simulink model "mrefrobotarm_modified_previous_y_previous_u_previous_ref_prepro"  (R2018b)
settings: Solver=FixedStepAuto  StartTime=0.0  StopTime=10  RelTol=1e-3  AbsTol=1e-6
undefined symbols (not defined in the file or in its folder): cc, options
libraries: neural x594, simulink x1
(part 16 of 22)

== system mrefrobotarm_modified_previous_y_previous_u_previous_ref_prepro/pre_0.00004/Layer 3/Delays 1 ==
  "p{3}" : Inport  PortDimensions=30
      mask Display: e = 0.06;c1 = [120 230 180]/255;c2 = ([120 230 180]+0)/(256+128);c3 = ([120 230 180]+128)/(256+128);patch([0 1 1 0],[0 0 1 1],c1);patch([0 1 1 1-e 1-e 0+e],[0 0 1 1-e 0+e 0+e],c2);patch([0 0 1 1-e 0+e 0+e],[0 1 1 1-e 1-e 0+e],c3);plot([0 1 1 0 0],[0 0 1 1 0]);
  mux : Mux  Inputs=1
      mask Display: e = 0.06;c1 = [120 150 230]/255;c2 = ([120 150 230]+0)/383;c3 = ([120 150 230]+128)/383;patch([0 1 1 0],[0 0 1 1],c1);patch([0 1 1 1-e 1-e 0+e],[0 0 1 1-e 0+e 0+e],c2);patch([0 0 1 1-e 0+e 0+e],[0 1 1 1-e 1-e 0+e],c3);plot([0 1 1 0 0],[0 0 1 1 0]);disp('Mux')
  "pd{3,2}" : Outport
      mask Display: e = 0.06;c1 = [120 230 180]/255;c2 = ([120 230 180]+0)/(256+128);c3 = ([120 230 180]+128)/(256+128);patch([0 1 1 0],[0 0 1 1],c1);patch([0 1 1 1-e 1-e 0+e],[0 0 1 1-e 0+e 0+e],c2);patch([0 0 1 1-e 0+e 0+e],[0 1 1 1-e 1-e 0+e],c3);plot([0 1 1 0 0],[0 0 1 1 0]);
  wires:
  "p{3}"/1 -> mux/1
  mux/1 -> "pd{3,2}"/1

== system mrefrobotarm_modified_previous_y_previous_u_previous_ref_prepro/pre_0.00004/Layer 3/LW{3,2} ==
  "ad{3,2}" : Inport  PortDimensions=30
      mask Display: e = 0.06;c1 = [120 230 180]/255;c2 = ([120 230 180]+0)/(256+128);c3 = ([120 230 180]+128)/(256+128);patch([0 1 1 0],[0 0 1 1],c1);patch([0 1 1 1-e 1-e 0+e],[0 0 1 1-e 0+e 0+e],c2);patch([0 0 1 1-e 0+e 0+e],[0 1 1 1-e 1-e 0+e],c3);plot([0 1 1 0 0],[0 0 1 1 0]);
  "IW{3,2}(1,:)'" : Constant  Value=[-0.12115323977208213024336913576917140744626522064208984375;0.1421645828481130913178986929779057390987873077392578125;0.2104360456092702891250922903054743073880672454833984375;-0.209627821379691436920467140225809998810291290283203125;0.399324974589913506139993160104495473206043243408203125;0.5108287033332643556349239588598720729351043701171875;-0.01755690203553068873265630145397153683006763458251953125;-0.398676925843608864763467636294080875813961029052734375;0.00184641474824170752355723124082942376844584941864013671875;0.267730388383461248569261670127161778509616851806640625;-0.2285341543329846292209595048916526138782501220703125;-0.14635003276886104917053899043821729719638824462890625;-0.290530902647844369024454636019072495400905609130859375;-0.18623054223144297480985187576152384281158447265625;-0.3816641765859636326041481879656203091144561767578125;0.422608587689044135071725349916960112750530242919921875;-0.50402602801203333360291480857995338737964630126953125;0.04787057638839231632488235845812596380710601806640625;0.26072024791618420014316370725282467901706695556640625;0.03130735790264956019957054422775399871170520782470703125;-0.184803625769296819836284839766449294984340667724609375;-0.07897098331966272144466501003989833407104015350341796875;0.318614464740402614228997890677419491112232208251953125;-0.32476411310026553902474688584334217011928558349609375;0.31226160654872237021351111252442933619022369384765625;0.08174671514652807891021524255847907625138759613037109375;-0.289500256123392085694234765469445846974849700927734375;-0.2644913786315357118184010687400586903095245361328125;0.06532576379320138848516563712109928019344806671142578125;0.088750906118596761817940432592877186834812164306640625]
      mask Display: e = 0.06;c1 = [120 150 230]/255;c2 = ([120 150 230]+0)/383;c3 = ([120 150 230]+128)/383;patch([0 1 1 0],[0 0 1 1],c1);patch([0 1 1 1-e 1-e 0+e],[0 0 1 1-e 0+e 0+e],c2);patch([0 0 1 1-e 0+e 0+e],[0 1 1 1-e 1-e 0+e],c3);plot([0 1 1 0 0],[0 0 1 1 0]);disp('weights');
  Mux : Mux  Inputs=1
      mask Display: e = 0.06;c1 = [120 150 230]/255;c2 = ([120 150 230]+0)/383;c3 = ([120 150 230]+128)/383;patch([0 1 1 0],[0 0 1 1],c1);patch([0 1 1 1-e 1-e 0+e],[0 0 1 1-e 0+e 0+e],c2);patch([0 0 1 1-e 0+e 0+e],[0 1 1 1-e 1-e 0+e],c3);plot([0 1 1 0 0],[0 0 1 1 0]);disp('Mux');
  dotprod1 : neural/Weight Functions/dotprod
  "lz{3,2}" : Outport
      mask Display: e = 0.06;c1 = [120 230 180]/255;c2 = ([120 230 180]+0)/(256+128);c3 = ([120 230 180]+128)/(256+128);patch([0 1 1 0],[0 0 1 1],c1);patch([0 1 1 1-e 1-e 0+e],[0 0 1 1-e 0+e 0+e],c2);patch([0 0 1 1-e 0+e 0+e],[0 1 1 1-e 1-e 0+e],c3);plot([0 1 1 0 0],[0 0 1 1 0]);
  wires:
  "IW{3,2}(1,:)'"/1 -> dotprod1/1
  "ad{3,2}"/1 -> dotprod1/2
  dotprod1/1 -> Mux/1
  Mux/1 -> "lz{3,2}"/1

== system mrefrobotarm_modified_previous_y_previous_u_previous_ref_prepro/pre_0.0001/Layer 1/Delays 1 ==
  "p{1}" : Inport  PortDimensions=10
      mask Display: e = 0.06;c1 = [120 230 180]/255;c2 = ([120 230 180]+0)/(256+128);c3 = ([120 230 180]+128)/(256+128);patch([0 1 1 0],[0 0 1 1],c1);patch([0 1 1 1-e 1-e 0+e],[0 0 1 1-e 0+e 0+e],c2);patch([0 0 1 1-e 0+e 0+e],[0 1 1 1-e 1-e 0+e],c3);plot([0 1 1 0 0],[0 0 1 1 0]);
  mux : Mux  Inputs=1
      mask Display: e = 0.06;c1 = [120 150 230]/255;c2 = ([120 150 230]+0)/383;c3 = ([120 150 230]+128)/383;patch([0 1 1 0],[0 0 1 1],c1);patch([0 1 1 1-e 1-e 0+e],[0 0 1 1-e 0+e 0+e],c2);patch([0 0 1 1-e 0+e 0+e],[0 1 1 1-e 1-e 0+e],c3);plot([0 1 1 0 0],[0 0 1 1 0]);disp('Mux')
  "pd{1,1}" : Outport
      mask Display: e = 0.06;c1 = [120 230 180]/255;c2 = ([120 230 180]+0)/(256+128);c3 = ([120 230 180]+128)/(256+128);patch([0 1 1 0],[0 0 1 1],c1);patch([0 1 1 1-e 1-e 0+e],[0 0 1 1-e 0+e 0+e],c2);patch([0 0 1 1-e 0+e 0+e],[0 1 1 1-e 1-e 0+e],c3);plot([0 1 1 0 0],[0 0 1 1 0]);
  wires:
  "p{1}"/1 -> mux/1
  mux/1 -> "pd{1,1}"/1

== system mrefrobotarm_modified_previous_y_previous_u_previous_ref_prepro/pre_0.0001/Layer 1/IW{1,1} ==
  "pd{1,1}" : Inport  PortDimensions=10
      mask Display: e = 0.06;c1 = [120 230 180]/255;c2 = ([120 230 180]+0)/(256+128);c3 = ([120 230 180]+128)/(256+128);patch([0 1 1 0],[0 0 1 1],c1);patch([0 1 1 1-e 1-e 0+e],[0 0 1 1-e 0+e 0+e],c2);patch([0 0 1 1-e 0+e 0+e],[0 1 1 1-e 1-e 0+e],c3);plot([0 1 1 0 0],[0 0 1 1 0]);
  "IW{1,1}(1,:)'" : Constant  Value=[0.48848188030832784267687429746729321777820587158203125;-0.50670985753113895189159165965975262224674224853515625;0.10409356491148090417819815911570913158357143402099609375;0.225809349826792404858366580810979939997196197509765625;0.4009865161841350555960161727853119373321533203125;0.169825092265467658680933027426362968981266021728515625;0.78830762047560887229025183842168189585208892822265625;0.8853776813051636995766102700144983828067779541015625;-1.267910607500292829996624277555383741855621337890625;-0.31884147881028657156576855413732118904590606689453125]
      mask Display: e = 0.06;c1 = [120 150 230]/255;c2 = ([120 150 230]+0)/383;c3 = ([120 150 230]+128)/383;patch([0 1 1 0],[0 0 1 1],c1);patch([0 1 1 1-e 1-e 0+e],[0 0 1 1-e 0+e 0+e],c2);patch([0 0 1 1-e 0+e 0+e],[0 1 1 1-e 1-e 0+e],c3);plot([0 1 1 0 0],[0 0 1 1 0]);disp('Weights');
  "IW{1,1}(10,:)'" : Constant  Value=[0.60982224497398618279220272597740404307842254638671875;-0.93656291188809603909248835407197475433349609375;0.0979830538632104619534146650039474479854106903076171875;-0.87957865814192859321707373965182341635227203369140625;-0.30231253806006563866759506709058769047260284423828125;0.199503786892032464184154605391086079180240631103515625;-1.1899431974826459867955463778343982994556427001953125;-0.03266430327928458721142845888607553206384181976318359375;0.3019162611871599732893400869215838611125946044921875;0.1610107886790740627791507222354994155466556549072265625]
      mask Display: e = 0.06;c1 = [120 150 230]/255;c2 = ([120 150 230]+0)/383;c3 = ([120 150 230]+128)/383;patch([0 1 1 0],[0 0 1 1],c1);patch([0 1 1 1-e 1-e 0+e],[0 0 1 1-e 0+e 0+e],c2);patch([0 0 1 1-e 0+e 0+e],[0 1 1 1-e 1-e 0+e],c3);plot([0 1 1 0 0],[0 0 1 1 0]);disp('Weights');
  "IW{1,1}(11,:)'" : Constant  Value=[0.43117720603294940051597450292319990694522857666015625;-1.1157191661762866363716284467955119907855987548828125;0.3922109909243991499039339032606221735477447509765625;-0.496959837462516540451673563438816927373409271240234375;0.01695143984838747008847548158883000724017620086669921875;1.3205255898856946839003967397729866206645965576171875;0.02046825294557734487010947077578748576343059539794921875;-0.346542077133276948952556040239869616925716400146484375;-0.87405349501553997182412558686337433755397796630859375;0.49868545376052519912946081603877246379852294921875]
      mask Display: e = 0.06;c1 = [120 150 230]/255;c2 = ([120 150 230]+0)/383;c3 = ([120 150 230]+128)/383;patch([0 1 1 0],[0 0 1 1],c1);patch([0 1 1 1-e 1-e 0+e],[0 0 1 1-e 0+e 0+e],c2);patch([0 0 1 1-e 0+e 0+e],[0 1 1 1-e 1-e 0+e],c3);plot([0 1 1 0 0],[0 0 1 1 0]);disp('Weights');
  "IW{1,1}(12,:)'" : Constant  Value=[-0.545805604712654268695359860430471599102020263671875;-0.65828716083673766146233674589893780648708343505859375;-0.04018956631550653357809466115213581360876560211181640625;0.06817452770580727239302376574414665810763835906982421875;-0.812439650403700586167587971431203186511993408203125;-0.15845568778963892153655024230829440057277679443359375;-0.345942575000688201658505249724839814007282257080078125;-0.1536078830084397217614622377368505112826824188232421875;-0.9507981209733535887806965547497384250164031982421875;-0.93008098611112532960731869025039486587047576904296875]
      mask Display: e = 0.06;c1 = [120 150 230]/255;c2 = ([120 150 230]+0)/383;c3 = ([120 150 230]+128)/383;patch([0 1 1 0],[0 0 1 1],c1);patch([0 1 1 1-e 1-e 0+e],[0 0 1 1-e 0+e 0+e],c2);patch([0 0 1 1-e 0+e 0+e],[0 1 1 1-e 1-e 0+e],c3);plot([0 1 1 0 0],[0 0 1 1 0]);disp('Weights');
  "IW{1,1}(13,:)'" : Constant  Value=[0.66295360405807157722080091843963600695133209228515625;-0.8938461691272043818656811708933673799037933349609375;-0.307383457603058740659207614953629672527313232421875;0.7696942151114913865939115567016415297985076904296875;-0.6424429227981693912852279026992619037628173828125;-0.88351184707840768606246228955569677054882049560546875;0.426220147155879691691637844996876083314418792724609375;-0.5581320405845280330225932630128227174282073974609375;0.313391024789088812330106748049729503691196441650390625;-0.273790918636316382706041849814937449991703033447265625]
      mask Display: e = 0.06;c1 = [120 150 230]/255;c2 = ([120 150 230]+0)/383;c3 = ([120 150 230]+128)/383;patch([0 1 1 0],[0 0 1 1],c1);patch([0 1 1 1-e 1-e 0+e],[0 0 1 1-e 0+e 0+e],c2);patch([0 0 1 1-e 0+e 0+e],[0 1 1 1-e 1-e 0+e],c3);plot([0 1 1 0 0],[0 0 1 1 0]);disp('Weights');
  "IW{1,1}(14,:)'" : Constant  Value=[-0.92662765081657616494936746676103211939334869384765625;-0.77592893914042460057345351742696948349475860595703125;-0.38812396597961573707635807295446284115314483642578125;-0.85245647876413166432740808886592276394367218017578125;-0.9446570653230501601882451723213307559490203857421875;-1.288106041851058147784669927204959094524383544921875;0.16689146233317309064858591227675788104534149169921875;0.2316131250010416142703917330436524935066699981689453125;-0.052082097249804192029554172904681763611733913421630859375;0.388945022452433175619290750546497292816638946533203125]
      mask Display: e = 0.06;c1 = [120 150 230]/255;c2 = ([120 150 230]+0)/383;c3 = ([120 150 230]+128)/383;patch([0 1 1 0],[0 0 1 1],c1);patch([0 1 1 1-e 1-e 0+e],[0 0 1 1-e 0+e 0+e],c2);patch([0 0 1 1-e 0+e 0+e],[0 1 1 1-e 1-e 0+e],c3);plot([0 1 1 0 0],[0 0 1 1 0]);disp('Weights');
  "IW{1,1}(15,:)'" : Constant  Value=[0.393002504312302658462385807069949805736541748046875;-0.91204255873710493585093672663788311183452606201171875;-0.6838111078302289147501369370729662477970123291015625;0.69939813890604252133442741978797130286693572998046875;0.1359188029727505242494345338855055160820484161376953125;1.6157726036601778307755239438847638666629791259765625;-0.5746204920280255645792522045667283236980438232421875;-1.0834603685301884556935192449600435793399810791015625;-1.6108799859154416811435339695890434086322784423828125;-0.6408546721886410058033334280480630695819854736328125]
      mask Display: e = 0.06;c1 = [120 150 230]/255;c2 = ([120 150 230]+0)/383;c3 = ([120 150 230]+128)/383;patch([0 1 1 0],[0 0 1 1],c1);patch([0 1 1 1-e 1-e 0+e],[0 0 1 1-e 0+e 0+e],c2);patch([0 0 1 1-e 0+e 0+e],[0 1 1 1-e 1-e 0+e],c3);plot([0 1 1 0 0],[0 0 1 1 0]);disp('Weights');
  "IW{1,1}(16,:)'" : Constant  Value=[-0.5822446766001101448040344621404074132442474365234375;-0.36869054704071613226545878205797635018825531005859375;-0.63677314866086887068519217791617847979068756103515625;0.362398212686899146017793782448279671370983123779296875;0.752496240116242720574746272177435457706451416015625;1.0345724771553974630222683117608539760112762451171875;-1.4227975354059168022757830840419046580791473388671875;0.76214623331916564463739405255182646214962005615234375;-0.71910385203646765006624264060519635677337646484375;-0.055712751883015505793839139414558303542435169219970703125]
      mask Display: e = 0.06;c1 = [120 150 230]/255;c2 = ([120 150 230]+0)/383;c3 = ([120 150 230]+128)/383;patch([0 1 1 0],[0 0 1 1],c1);patch([0 1 1 1-e 1-e 0+e],[0 0 1 1-e 0+e 0+e],c2);patch([0 0 1 1-e 0+e 0+e],[0 1 1 1-e 1-e 0+e],c3);plot([0 1 1 0 0],[0 0 1 1 0]);disp('Weights');
  "IW{1,1}(17,:)'" : Constant  Value=[0.38424423751284553230078699925797991454601287841796875;-0.526966471090468235871639990364201366901397705078125;-0.226879550264598328634946255988324992358684539794921875;-0.8968543944114590882321635945118032395839691162109375;1.1127555884072781733351575894630514085292816162109375;0.27880392633728001694493059403612278401851654052734375;-1.5071767823827830756755474794772453606128692626953125;-0.55771359207759851894792291204794310033321380615234375;-0.399993902113242316698205058855819515883922576904296875;0.5331078302431866422494977086898870766162872314453125]
      mask Display: e = 0.06;c1 = [120 150 230]/255;c2 = ([120 150 230]+0)/383;c3 = ([120 150 230]+128)/383;patch([0 1 1 0],[0 0 1 1],c1);patch([0 1 1 1-e 1-e 0+e],[0 0 1 1-e 0+e 0+e],c2);patch([0 0 1 1-e 0+e 0+e],[0 1 1 1-e 1-e 0+e],c3);plot([0 1 1 0 0],[0 0 1 1 0]);disp('Weights');
  "IW{1,1}(18,:)'" : Constant  Value=[-0.86072504364026924950081820497871376574039459228515625;0.105831858781591015006284806077019311487674713134765625;0.78501692422073732213760877129971049726009368896484375;-0.526503490628730030920223725843243300914764404296875;-1.60365143543755639399250867427326738834381103515625;1.704772031990960723391026476747356355190277099609375;0.182640145479193771738124496550881303846836090087890625;0.56937911605091195976768858599825762212276458740234375;-0.615288271359693883510999512509442865848541259765625;0.1801509164855399358629028938594274222850799560546875]
      mask Display: e = 0.06;c1 = [120 150 230]/255;c2 = ([120 150 230]+0)/383;c3 = ([120 150 230]+128)/383;patch([0 1 1 0],[0 0 1 1],c1);patch([0 1 1 1-e 1-e 0+e],[0 0 1 1-e 0+e 0+e],c2);patch([0 0 1 1-e 0+e 0+e],[0 1 1 1-e 1-e 0+e],c3);plot([0 1 1 0 0],[0 0 1 1 0]);disp('Weights');
  "IW{1,1}(19,:)'" : Constant  Value=[0.9433236423230793032956853494397364556789398193359375;-0.41651660729159178941927166306413710117340087890625;0.47987865442477628530326683176099322736263275146484375;0.9705276609565613998853450539172627031803131103515625;-0.63524682091880702028419136695447377860546112060546875;-0.16206036147496460930739203831763006746768951416015625;0.79611869556153058713476866614655591547489166259765625;0.998942204364766439539380371570587158203125;-0.354438797782582193374167900401516817510128021240234375;-0.298955544274303319784991117558092810213565826416015625]
      mask Display: e = 0.06;c1 = [120 150 230]/255;c2 = ([120 150 230]+0)/383;c3 = ([120 150 230]+128)/383;patch([0 1 1 0],[0 0 1 1],c1);patch([0 1 1 1-e 1-e 0+e],[0 0 1 1-e 0+e 0+e],c2);patch([0 0 1 1-e 0+e 0+e],[0 1 1 1-e 1-e 0+e],c3);plot([0 1 1 0 0],[0 0 1 1 0]);disp('Weights');
  "IW{1,1}(2,:)'" : Constant  Value=[-0.7683446590382312368916473133140243589878082275390625;0.440364164479861763812351682645385153591632843017578125;0.7610214354865878494393882647273130714893341064453125;-0.436521421785640406643125288610463030636310577392578125;0.03200275340574865179377184176701121032238006591796875;-1.4094170015904217141411436386988498270511627197265625;1.0032431537181150105197957600466907024383544921875;0.53363762883434684436423367515089921653270721435546875;0.7394109627995908429198834710405208170413970947265625;-0.28852296259112908405342068363097496330738067626953125]
      mask Display: e = 0.06;c1 = [120 150 230]/255;c2 = ([120 150 230]+0)/383;c3 = ([120 150 230]+128)/383;patch([0 1 1 0],[0 0 1 1],c1);patch([0 1 1 1-e 1-e 0+e],[0 0 1 1-e 0+e 0+e],c2);patch([0 0 1 1-e 0+e 0+e],[0 1 1 1-e 1-e 0+e],c3);plot([0 1 1 0 0],[0 0 1 1 0]);disp('Weights');
  "IW{1,1}(20,:)'" : Constant  Value=[-0.7009040048614483264799446260440163314342498779296875;0.94369274324384655461273041510139591991901397705078125;-0.8314556402944646151809138245880603790283203125;-0.332716420599462769924770100260502658784389495849609375;-1.60251138267192327901966564240865409374237060546875;2.1342861071012517726330770528875291347503662109375;-0.57596256925930011671965758068836294114589691162109375;-0.70435812021294907925295092354645021259784698486328125;-0.595064456252060836050077341496944427490234375;-0.4644145978565792365344577774521894752979278564453125]
      mask Display: e = 0.06;c1 = [120 150 230]/255;c2 = ([120 150 230]+0)/383;c3 = ([120 150 230]+128)/383;patch([0 1 1 0],[0 0 1 1],c1);patch([0 1 1 1-e 1-e 0+e],[0 0 1 1-e 0+e 0+e],c2);patch([0 0 1 1-e 0+e 0+e],[0 1 1 1-e 1-e 0+e],c3);plot([0 1 1 0 0],[0 0 1 1 0]);disp('Weights');
  "IW{1,1}(21,:)'" : Constant  Value=[0.37115364933432604122032216764637269079685211181640625;0.912598488166298071888604681589640676975250244140625;-0.94118622538714247216518060668022371828556060791015625;0.327716496180934069304413469581049866974353790283203125;-0.7991183749965913296620101391454227268695831298828125;1.6142260875824039345616256468929350376129150390625;-1.3204976180473380065194533017347566783428192138671875;-0.51577295266080180891066220283391885459423065185546875;0.390741506230239565855555383677710779011249542236328125;-0.2408874449165481212986605896730907261371612548828125]
      mask Display: e = 0.06;c1 = [120 150 230]/255;c2 = ([120 150 230]+0)/383;c3 = ([120 150 230]+128)/383;patch([0 1 1 0],[0 0 1 1],c1);patch([0 1 1 1-e 1-e 0+e],[0 0 1 1-e 0+e 0+e],c2);patch([0 0 1 1-e 0+e 0+e],[0 1 1 1-e 1-e 0+e],c3);plot([0 1 1 0 0],[0 0 1 1 0]);disp('Weights');
  "IW{1,1}(22,:)'" : Constant  Value=[-0.890358740836964646092610564664937555789947509765625;-0.59720930092109603126715455800876952707767486572265625;-0.2401630259369448017192638644701219163835048675537109375;0.84055966717644092778272124633076600730419158935546875;0.7463616014768483797325870909844525158405303955078125;-0.059133371953366042905742006041691638529300689697265625;0.254524340337156596003609365652664564549922943115234375;-1.466536613227618079946523721446283161640167236328125;-0.2252389171432715719856076930227573029696941375732421875;0.3900174608220841054873062603292055428028106689453125]
      mask Display: e = 0.06;c1 = [120 150 230]/255;c2 = ([120 150 230]+0)/383;c3 = ([120 150 230]+128)/383;patch([0 1 1 0],[0 0 1 1],c1);patch([0 1 1 1-e 1-e 0+e],[0 0 1 1-e 0+e 0+e],c2);patch([0 0 1 1-e 0+e 0+e],[0 1 1 1-e 1-e 0+e],c3);plot([0 1 1 0 0],[0 0 1 1 0]);disp('Weights');
  "IW{1,1}(23,:)'" : Constant  Value=[-0.250099872437748282916203379500075243413448333740234375;-0.6330298234133120427458152335020713508129119873046875;0.05984102964771779997743550438826787285506725311279296875;0.52289087035782533252614712182548828423023223876953125;1.23261149620844623342463819426484405994415283203125;-0.1076436076036490219198782369858236052095890045166015625;-0.56761274851062382129640582206775434315204620361328125;-0.63316245325842590574438872863538563251495361328125;0.3660360442242700518278297749930061399936676025390625;-1.44190677819273815885026124306023120880126953125]
      mask Display: e = 0.06;c1 = [120 150 230]/255;c2 = ([120 150 230]+0)/383;c3 = ([120 150 230]+128)/383;patch([0 1 1 0],[0 0 1 1],c1);patch([0 1 1 1-e 1-e 0+e],[0 0 1 1-e 0+e 0+e],c2);patch([0 0 1 1-e 0+e 0+e],[0 1 1 1-e 1-e 0+e],c3);plot([0 1 1 0 0],[0 0 1 1 0]);disp('Weights');
  "IW{1,1}(24,:)'" : Constant  Value=[0.28011911085527263498562433596816845238208770751953125;-1.37130107604782391916842243517749011516571044921875;0.888718950676372632102584248059429228305816650390625;-0.11584040208703906549292383942884043790400028228759765625;-1.1677404204668813125778115136199630796909332275390625;0.6389640316349780579940897951018996536731719970703125;-0.2106874349715198435628593642832129262387752532958984375;0.41130394093588173998199408742948435246944427490234375;0.65910753951993650279206349296146072447299957275390625;0.70223307242311838738402229864732362329959869384765625]
      mask Display: e = 0.06;c1 = [120 150 230]/255;c2 = ([120 150 230]+0)/383;c3 = ([120 150 230]+128)/383;patch([0 1 1 0],[0 0 1 1],c1);patch([0 1 1 1-e 1-e 0+e],[0 0 1 1-e 0+e 0+e],c2);patch([0 0 1 1-e 0+e 0+e],[0 1 1 1-e 1-e 0+e],c3);plot([0 1 1 0 0],[0 0 1 1 0]);disp('Weights');
  "IW{1,1}(25,:)'" : Constant  Value=[0.11988820609216861712287283125988324172794818878173828125;0.68913309953840506949518385226838290691375732421875;-0.03502681873182401928179530159468413330614566802978515625;0.722591710239250506475627844338305294513702392578125;-0.5421905713423977868359315834823064506053924560546875;-0.74942099904761028117405885495827533304691314697265625;0.0132182290416811738797964181912902859039604663848876953125;0.63444274100397579640997491878806613385677337646484375;1.134709273244190352869509297306649386882781982421875;1.12762948313575517289564231759868562221527099609375]
      mask Display: e = 0.06;c1 = [120 150 230]/255;c2 = ([120 150 230]+0)/383;c3 = ([120 150 230]+128)/383;patch([0 1 1 0],[0 0 1 1],c1);patch([0 1 1 1-e 1-e 0+e],[0 0 1 1-e 0+e 0+e],c2);patch([0 0 1 1-e 0+e 0+e],[0 1 1 1-e 1-e 0+e],c3);plot([0 1 1 0 0],[0 0 1 1 0]);disp('Weights');
  "IW{1,1}(26,:)'" : Constant  Value=[0.82218785896144519487194202156388200819492340087890625;-0.0384600880471717143649357240065000951290130615234375;0.81635902356652056965913288877345621585845947265625;-0.651885940487107351515305708744563162326812744140625;0.296474753586223993551129751722328364849090576171875;-0.01452889102339892379855967874391353689134120941162109375;-0.1303808217281205161786061808015801943838596343994140625;0.2389865392911683372734188424146850593388080596923828125;-0.84025197912634297381373471580445766448974609375;0.597782619879347887348330914392136037349700927734375]
      mask Display: e = 0.06;c1 = [120 150 230]/255;c2 = ([120 150 230]+0)/383;c3 = ([120 150 230]+128)/383;patch([0 1 1 0],[0 0 1 1],c1);patch([0 1 1 1-e 1-e 0+e],[0 0 1 1-e 0+e 0+e],c2);patch([0 0 1 1-e 0+e 0+e],[0 1 1 1-e 1-e 0+e],c3);plot([0 1 1 0 0],[0 0 1 1 0]);disp('Weights');
  "IW{1,1}(27,:)'" : Constant  Value=[0.322839363440056204002104323080857284367084503173828125;1.131809766019331586761609287350438535213470458984375;0.3754425774053189446277656315942294895648956298828125;-0.39291904514102193868296808432205580174922943115234375;0.50443587321623806207782081401092000305652618408203125;0.26038106338422928320852633987669833004474639892578125;0.363507168221817666964312820709892548620700836181640625;-1.035154241252492557379127902095206081867218017578125;0.7991545461858493570872497002710588276386260986328125;0.32930271931210575164783449508831836283206939697265625]
      mask Display: e = 0.06;c1 = [120 150 230]/255;c2 = ([120 150 230]+0)/383;c3 = ([120 150 230]+128)/383;patch([0 1 1 0],[0 0 1 1],c1);patch([0 1 1 1-e 1-e 0+e],[0 0 1 1-e 0+e 0+e],c2);patch([0 0 1 1-e 0+e 0+e],[0 1 1 1-e 1-e 0+e],c3);plot([0 1 1 0 0],[0 0 1 1 0]);disp('Weights');
  "IW{1,1}(28,:)'" : Constant  Value=[0.0389583474877909508027329366086632944643497467041015625;0.4096437612245027448665268821059726178646087646484375;0.25546673540113939981921475919079966843128204345703125;0.662541768319801160913584681111387908458709716796875;0.52555753194784615711654396363883279263973236083984375;-1.4119576189336544569385978320497088134288787841796875;1.1993812385580222557024399065994657576084136962890625;0.590564151836458162136977989575825631618499755859375;1.0111070041476306613503766129724681377410888671875;0.2252881008519034555792615037717041559517383575439453125]
      mask Display: e = 0.06;c1 = [120 150 230]/255;c2 = ([120 150 230]+0)/383;c3 = ([120 150 230]+128)/383;patch([0 1 1 0],[0 0 1 1],c1);patch([0 1 1 1-e 1-e 0+e],[0 0 1 1-e 0+e 0+e],c2);patch([0 0 1 1-e 0+e 0+e],[0 1 1 1-e 1-e 0+e],c3);plot([0 1 1 0 0],[0 0 1 1 0]);disp('Weights');
  "IW{1,1}(29,:)'" : Constant  Value=[-0.6747496255076617099888380835182033479213714599609375;1.3118944028766446052713945391587913036346435546875;-0.1658332381289283896652619887390756048262119293212890625;0.35876508635926551704642406548373401165008544921875;0.2155241399386029765850025796680711209774017333984375;-1.194955820227538101363506939378567039966583251953125;0.68359442823319493953704295563511550426483154296875;0.80661029192979316615463858397561125457286834716796875;-0.29614206805014398060649227772955782711505889892578125;-0.754145806357484627113763053785078227519989013671875]
      mask Display: e = 0.06;c1 = [120 150 230]/255;c2 = ([120 150 230]+0)/383;c3 = ([120 150 230]+128)/383;patch([0 1 1 0],[0 0 1 1],c1);patch([0 1 1 1-e 1-e 0+e],[0 0 1 1-e 0+e 0+e],c2);patch([0 0 1 1-e 0+e 0+e],[0 1 1 1-e 1-e 0+e],c3);plot([0 1 1 0 0],[0 0 1 1 0]);disp('Weights');
  "IW{1,1}(3,:)'" : Constant  Value=[0.8150004602918989871085386766935698688030242919921875;-0.34847040275175500401161343688727356493473052978515625;0.63045392616037199129408463704749010503292083740234375;-0.33417427628333518097036858307546935975551605224609375;0.6718122097003045301022439161897636950016021728515625;0.09543688997760142733728372377299820072948932647705078125;-0.60462897982715746447723859091638587415218353271484375;1.008487393039244839343382409424521028995513916015625;-0.5163466201618673867557163248420692980289459228515625;-0.6113547201688864785040777860558591783046722412109375]
      mask Display: e = 0.06;c1 = [120 150 230]/255;c2 = ([120 150 230]+0)/383;c3 = ([120 150 230]+128)/383;patch([0 1 1 0],[0 0 1 1],c1);patch([0 1 1 1-e 1-e 0+e],[0 0 1 1-e 0+e 0+e],c2);patch([0 0 1 1-e 0+e 0+e],[0 1 1 1-e 1-e 0+e],c3);plot([0 1 1 0 0],[0 0 1 1 0]);disp('Weights');
  "IW{1,1}(30,:)'" : Constant  Value=[0.8587818165224347932706905339728109538555145263671875;-1.0096021379255006866770827400614507496356964111328125;0.95949982654104581936138629316701553761959075927734375;0.36408533279713850561165600083768367767333984375;-0.1268926435739388958179318933616741560399532318115234375;-0.0164013498249012852625572378428842057473957538604736328125;0.53658117729785093086292135922121815383434295654296875;0.166459034803973338068061593730817548930644989013671875;-0.0215228741508084742140027856294182129204273223876953125;0.389859014857539543097431078422232531011104583740234375]
      mask Display: e = 0.06;c1 = [120 150 230]/255;c2 = ([120 150 230]+0)/383;c3 = ([120 150 230]+128)/383;patch([0 1 1 0],[0 0 1 1],c1);patch([0 1 1 1-e 1-e 0+e],[0 0 1 1-e 0+e 0+e],c2);patch([0 0 1 1-e 0+e 0+e],[0 1 1 1-e 1-e 0+e],c3);plot([0 1 1 0 0],[0 0 1 1 0]);disp('Weights');
  "IW{1,1}(4,:)'" : Constant  Value=[0.58046682397663096342199651189730502665042877197265625;0.1815192205135983949393363445778959430754184722900390625;-1.0009575506117069920719586662016808986663818359375;0.334339595964117164417217509253532625734806060791015625;1.1823138222933609053910686270683072507381439208984375;-0.434943633467452850371870454182499088346958160400390625;-0.09557509376208507545502612856580526567995548248291015625;-0.6066544242368416828270483165397308766841888427734375;-0.2045378661215495885716819657318410463631153106689453125;-0.68271027997290556488252377675962634384632110595703125]
      mask Display: e = 0.06;c1 = [120 150 230]/255;c2 = ([120 150 230]+0)/383;c3 = ([120 150 230]+128)/383;patch([0 1 1 0],[0 0 1 1],c1);patch([0 1 1 1-e 1-e 0+e],[0 0 1 1-e 0+e 0+e],c2);patch([0 0 1 1-e 0+e 0+e],[0 1 1 1-e 1-e 0+e],c3);plot([0 1 1 0 0],[0 0 1 1 0]);disp('Weights');
  "IW{1,1}(5,:)'" : Constant  Value=[0.10629747717312322541349800530952052213251590728759765625;-0.84108605713199546816127849524491466581821441650390625;0.12139453176720162164148320016465731896460056304931640625;0.42223751015776922468347720496240071952342987060546875;0.00736402021357632739773091401502824737690389156341552734375;1.282734174894848866443908264045603573322296142578125;-1.1538976775545364272801407423685304820537567138671875;-0.61500743201550422956103147953399457037448883056640625;0.217958916005971559126663805727730505168437957763671875;0.38956643884839914360185275654657743871212005615234375]
      mask Display: e = 0.06;c1 = [120 150 230]/255;c2 = ([120 150 230]+0)/383;c3 = ([120 150 230]+128)/383;patch([0 1 1 0],[0 0 1 1],c1);patch([0 1 1 1-e 1-e 0+e],[0 0 1 1-e 0+e 0+e],c2);patch([0 0 1 1-e 0+e 0+e],[0 1 1 1-e 1-e 0+e],c3);plot([0 1 1 0 0],[0 0 1 1 0]);disp('Weights');
  "IW{1,1}(6,:)'" : Constant  Value=[-0.833627122224390060267751323408447206020355224609375;0.5263117082043813343972260554437525570392608642578125;-0.067346872473442564999146497939364053308963775634765625;-0.257850604331755162146322390981367789208889007568359375;-1.2431995202965449021093036208185367286205291748046875;0.72120351129655180244526491151191294193267822265625;-0.4502658828630419218796987479436211287975311279296875;0.92784874989719856586134483222849667072296142578125;0.07911816128165040373776406568140373565256595611572265625;-0.7844562790982581024223918575444258749485015869140625]
      mask Display: e = 0.06;c1 = [120 150 230]/255;c2 = ([120 150 230]+0)/383;c3 = ([120 150 230]+128)/383;patch([0 1 1 0],[0 0 1 1],c1);patch([0 1 1 1-e 1-e 0+e],[0 0 1 1-e 0+e 0+e],c2);patch([0 0 1 1-e 0+e 0+e],[0 1 1 1-e 1-e 0+e],c3);plot([0 1 1 0 0],[0 0 1 1 0]);disp('Weights');
  "IW{1,1}(7,:)'" : Constant  Value=[-0.32835795606422524262058004751452244818210601806640625;-0.05269374910068967687859498028046800754964351654052734375;-0.76875822875495447572546936498838476836681365966796875;-0.47846308607651655275816438006586395204067230224609375;-0.054304399688376470134443252391065470874309539794921875;1.496008234749194532042793071013875305652618408203125;-0.3880246479458036024112743689329363405704498291015625;-0.94214666805871549737361192455864511430263519287109375;-0.97222759007928616359350826314766891300678253173828125;-0.68949209064189975748604410910047590732574462890625]
      mask Display: e = 0.06;c1 = [120 150 230]/255;c2 = ([120 150 230]+0)/383;c3 = ([120 150 230]+128)/383;patch([0 1 1 0],[0 0 1 1],c1);patch([0 1 1 1-e 1-e 0+e],[0 0 1 1-e 0+e 0+e],c2);patch([0 0 1 1-e 0+e 0+e],[0 1 1 1-e 1-e 0+e],c3);plot([0 1 1 0 0],[0 0 1 1 0]);disp('Weights');
  "IW{1,1}(8,:)'" : Constant  Value=[0.6236654834490813481551185759599320590496063232421875;-0.2727650501540013205925561123876832425594329833984375;-1.4467382553933847422200642540701664984226226806640625;0.172907217405822433153872452749055810272693634033203125;-0.8126924725893263090625850963988341391086578369140625;0.037315711557900040074020608926730346865952014923095703125;-0.227299739498888764277495511123561300337314605712890625;-0.2320672591109949334242656959759187884628772735595703125;-0.6857151945679333948646672070026397705078125;-0.53385387713694443245771026340662501752376556396484375]
      mask Display: e = 0.06;c1 = [120 150 230]/255;c2 = ([120 150 230]+0)/383;c3 = ([120 150 230]+128)/383;patch([0 1 1 0],[0 0 1 1],c1);patch([0 1 1 1-e 1-e 0+e],[0 0 1 1-e 0+e 0+e],c2);patch([0 0 1 1-e 0+e 0+e],[0 1 1 1-e 1-e 0+e],c3);plot([0 1 1 0 0],[0 0 1 1 0]);disp('Weights');
  "IW{1,1}(9,:)'" : Constant  Value=[-0.831935606778020808604878766345791518688201904296875;0.87171445109504308579317921612528152763843536376953125;0.1359169104653441539909408675157465040683746337890625;0.3692161841467973548702730113291181623935699462890625;1.2677272948705766708599185221828520298004150390625;-0.9225841266587584410530098466551862657070159912109375;-0.00602532389048794116137575116454172530211508274078369140625;-0.7169304580796158621325275817071087658405303955078125;0.93660500678837854682257102467701770365238189697265625;-0.0678121476613877394168383716532844118773937225341796875]
      mask Display: e = 0.06;c1 = [120 150 230]/255;c2 = ([120 150 230]+0)/383;c3 = ([120 150 230]+128)/383;patch([0 1 1 0],[0 0 1 1],c1);patch([0 1 1 1-e 1-e 0+e],[0 0 1 1-e 0+e 0+e],c2);patch([0 0 1 1-e 0+e 0+e],[0 1 1 1-e 1-e 0+e],c3);plot([0 1 1 0 0],[0 0 1 1 0]);disp('Weights');
  Mux : Mux  Inputs=30
      mask Display: e = 0.06;c1 = [120 150 230]/255;c2 = ([120 150 230]+0)/383;c3 = ([120 150 230]+128)/383;patch([0 1 1 0],[0 0 1 1],c1);patch([0 1 1 1-e 1-e 0+e],[0 0 1 1-e 0+e 0+e],c2);patch([0 0 1 1-e 0+e 0+e],[0 1 1 1-e 1-e 0+e],c3);plot([0 1 1 0 0],[0 0 1 1 0]);disp('Mux');
  dotprod{1..30} (30 alike) : neural/Weight Functions/dotprod
  "iz{1,1}" : Outport
      mask Display: e = 0.06;c1 = [120 230 180]/255;c2 = ([120 230 180]+0)/(256+128);c3 = ([120 230 180]+128)/(256+128);patch([0 1 1 0],[0 0 1 1],c1);patch([0 1 1 1-e 1-e 0+e],[0 0 1 1-e 0+e 0+e],c2);patch([0 0 1 1-e 0+e 0+e],[0 1 1 1-e 1-e 0+e],c3);plot([0 1 1 0 0],[0 0 1 1 0]);
  wires:
  "IW{1,1}(1,:)'"/1 -> dotprod1/1
  "pd{1,1}"/1 -> dotprod1/2, dotprod2/2, dotprod3/2, dotprod4/2, dotprod5/2, dotprod6/2, dotprod7/2, dotprod8/2, dotprod9/2, dotprod10/2, dotprod11/2, dotprod12/2, dotprod13/2, dotprod14/2, dotprod15/2, dotprod16/2, dotprod17/2, dotprod18/2, dotprod19/2, dotprod20/2, dotprod21/2, dotprod22/2, dotprod23/2, dotprod24/2, dotprod25/2, dotprod26/2, dotprod27/2, dotprod28/2, dotprod29/2, dotprod30/2
  dotprod1/1 -> Mux/1
  "IW{1,1}(2,:)'"/1 -> dotprod2/1
  dotprod2/1 -> Mux/2
  "IW{1,1}(3,:)'"/1 -> dotprod3/1
  dotprod3/1 -> Mux/3
  "IW{1,1}(4,:)'"/1 -> dotprod4/1
  dotprod4/1 -> Mux/4
  "IW{1,1}(5,:)'"/1 -> dotprod5/1
  dotprod5/1 -> Mux/5
  "IW{1,1}(6,:)'"/1 -> dotprod6/1
  dotprod6/1 -> Mux/6
  "IW{1,1}(7,:)'"/1 -> dotprod7/1
  dotprod7/1 -> Mux/7
  "IW{1,1}(8,:)'"/1 -> dotprod8/1
  dotprod8/1 -> Mux/8
  "IW{1,1}(9,:)'"/1 -> dotprod9/1
  dotprod9/1 -> Mux/9
  "IW{1,1}(10,:)'"/1 -> dotprod10/1
  dotprod10/1 -> Mux/10
  "IW{1,1}(11,:)'"/1 -> dotprod11/1
  dotprod11/1 -> Mux/11
  "IW{1,1}(12,:)'"/1 -> dotprod12/1
  dotprod12/1 -> Mux/12
  "IW{1,1}(13,:)'"/1 -> dotprod13/1
  dotprod13/1 -> Mux/13
  "IW{1,1}(14,:)'"/1 -> dotprod14/1
  dotprod14/1 -> Mux/14
  "IW{1,1}(15,:)'"/1 -> dotprod15/1
  dotprod15/1 -> Mux/15
  "IW{1,1}(16,:)'"/1 -> dotprod16/1
  dotprod16/1 -> Mux/16
  "IW{1,1}(17,:)'"/1 -> dotprod17/1
  dotprod17/1 -> Mux/17
  "IW{1,1}(18,:)'"/1 -> dotprod18/1
  dotprod18/1 -> Mux/18
  "IW{1,1}(19,:)'"/1 -> dotprod19/1
  dotprod19/1 -> Mux/19
  "IW{1,1}(20,:)'"/1 -> dotprod20/1
  dotprod20/1 -> Mux/20
  "IW{1,1}(21,:)'"/1 -> dotprod21/1
  dotprod21/1 -> Mux/21
  "IW{1,1}(22,:)'"/1 -> dotprod22/1
  dotprod22/1 -> Mux/22
  "IW{1,1}(23,:)'"/1 -> dotprod23/1
  dotprod23/1 -> Mux/23
  "IW{1,1}(24,:)'"/1 -> dotprod24/1
  dotprod24/1 -> Mux/24
  "IW{1,1}(25,:)'"/1 -> dotprod25/1
  dotprod25/1 -> Mux/25
  "IW{1,1}(26,:)'"/1 -> dotprod26/1
  dotprod26/1 -> Mux/26
  "IW{1,1}(27,:)'"/1 -> dotprod27/1
  dotprod27/1 -> Mux/27
  "IW{1,1}(28,:)'"/1 -> dotprod28/1
  dotprod28/1 -> Mux/28
  "IW{1,1}(29,:)'"/1 -> dotprod29/1
  dotprod29/1 -> Mux/29
  "IW{1,1}(30,:)'"/1 -> dotprod30/1
  dotprod30/1 -> Mux/30
  Mux/1 -> "iz{1,1}"/1

== system mrefrobotarm_modified_previous_y_previous_u_previous_ref_prepro/pre_0.0001/Layer 2/Delays 1 ==
  "p{2}" : Inport  PortDimensions=30
      mask Display: e = 0.06;c1 = [120 230 180]/255;c2 = ([120 230 180]+0)/(256+128);c3 = ([120 230 180]+128)/(256+128);patch([0 1 1 0],[0 0 1 1],c1);patch([0 1 1 1-e 1-e 0+e],[0 0 1 1-e 0+e 0+e],c2);patch([0 0 1 1-e 0+e 0+e],[0 1 1 1-e 1-e 0+e],c3);plot([0 1 1 0 0],[0 0 1 1 0]);
  mux : Mux  Inputs=1
      mask Display: e = 0.06;c1 = [120 150 230]/255;c2 = ([120 150 230]+0)/383;c3 = ([120 150 230]+128)/383;patch([0 1 1 0],[0 0 1 1],c1);patch([0 1 1 1-e 1-e 0+e],[0 0 1 1-e 0+e 0+e],c2);patch([0 0 1 1-e 0+e 0+e],[0 1 1 1-e 1-e 0+e],c3);plot([0 1 1 0 0],[0 0 1 1 0]);disp('Mux')
  "pd{2,1}" : Outport
      mask Display: e = 0.06;c1 = [120 230 180]/255;c2 = ([120 230 180]+0)/(256+128);c3 = ([120 230 180]+128)/(256+128);patch([0 1 1 0],[0 0 1 1],c1);patch([0 1 1 1-e 1-e 0+e],[0 0 1 1-e 0+e 0+e],c2);patch([0 0 1 1-e 0+e 0+e],[0 1 1 1-e 1-e 0+e],c3);plot([0 1 1 0 0],[0 0 1 1 0]);
  wires:
  "p{2}"/1 -> mux/1
  mux/1 -> "pd{2,1}"/1
